simulink model "TempControlExperiment"  (R2016a)
settings: Solver=FixedStepDiscrete  StartTime=0.0  StopTime=inf  FixedStep=1  RelTol=1e-3
libraries: simulink x7, EEE481Arduino x3
settings Model: ExtModeTrigDuration=2  Creator=rsjoshi1  LastModifiedBy=rsjoshi1
settings OptimizationCC: OptimizeModelRefInitCode=on  LifeSpan=Inf  MaxStackSize=64
settings HardwareCC: ProdBitPerPointer=32  ProdLargestAtomicInteger=Long  ProdLargestAtomicFloat=Double  ProdWordSize=32  ProdHWDeviceType=ARM Compatible->ARM Cortex
settings RTWCC: SystemTargetFile=ert.tlc  HardwareBoard=Arduino Due  TemplateMakefile=ert_default_tmf  GenerateReport=on  Toolchain=Arduino ARM v1.6.1  BuildConfiguration=Faster Runs  IncludeHyperlinkInReport=on  LaunchReport=on  GenerateTraceInfo=on  GenerateTraceReport=on  GenerateTraceReportSl=on  GenerateTraceReportSf=on  GenerateTraceReportEml=on
settings CodeAppCC: ForceParamTrailComments=on  IgnoreCustomStorageClasses=off  OperatorAnnotations=on  SimulinkDataObjDesc=on  SFDataObjDesc=on  MATLABFcnDesc=on  InsertBlockDesc=on  MATLABSourceComments=on
settings ERTTargetCC: SupportContinuousTime=on  SupportVariableSizeSignals=on

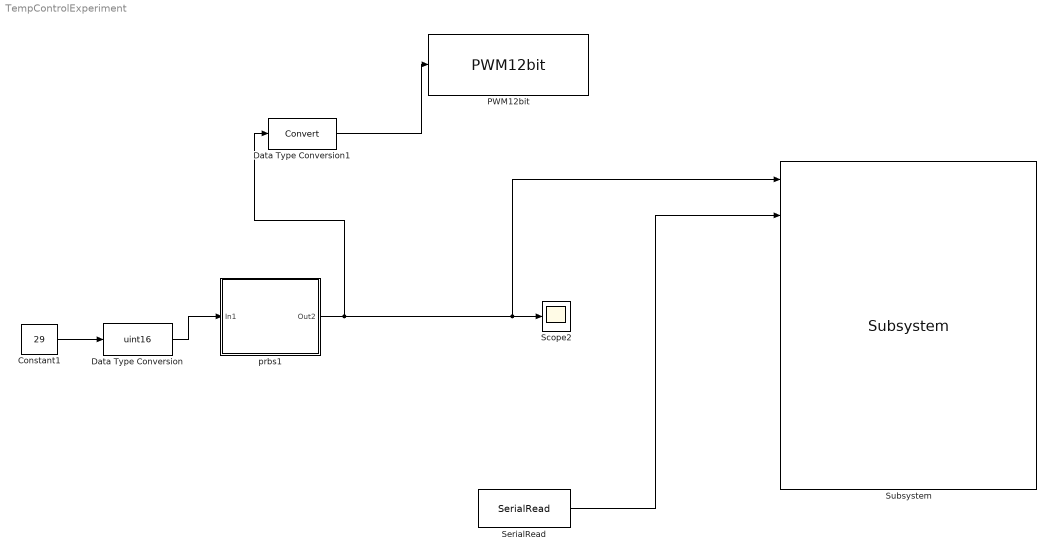
== system TempControlExperiment ==
  Constant1 : Constant  Value=29  OutDataTypeStr=double  SampleTime=1
  Data Type Conversion : DataTypeConversion  OutDataTypeStr=uint16
  Data Type Conversion1 : DataTypeConversion
  PWM12bit : EEE481Arduino/PWM12bit  PwmPort=8
  Scope2 : Scope
  SerialRead : EEE481Arduino/SerialRead  serialNum=2  Ts=1
  Subsystem : EEE481Arduino/Subsystem  Tsa=1  rate=0
  prbs1 : Subsystem
  wires:
  prbs1/1(Out2) -> Data Type Conversion1/1, Subsystem/1, Scope2/1
  Constant1/1 -> Data Type Conversion/1
  Data Type Conversion/1 -> prbs1/1(In1)
  SerialRead/1 -> Subsystem/2
  Data Type Conversion1/1 -> PWM12bit/1

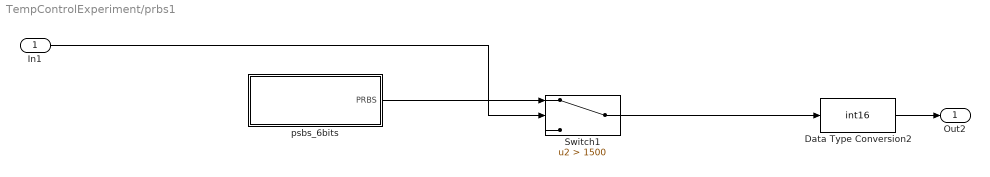
== system TempControlExperiment/prbs1 ==
  In1 : Inport
  Data Type Conversion2 : DataTypeConversion  OutDataTypeStr=int16
  Switch1 : Switch  Criteria=u2 > Threshold  Threshold=1500
  psbs_6bits : Subsystem  mask(PRBS with 8 shift registers){T=-1, Tsw=200, Lz=12000, Lv=60, Nc=100}
      mask prompts: T "Sample Time (s)"; Tsw "Time to switch (s)"; Lz "Leading Zeros (s)"; Lv "Switching Levels"; Nc "Number of Cycles"
      mask help:
      | Creates a PRBS signal using 6 shift registers.
      |     *Time to switch (Tsw) must be an integer multiple of Sample Time (T).
      |     *Leading zeros specify how long the PRBS will be zero, in seconds, before the levels begin shifting.
      |     *Level is the amplitude of the desired PRBS signal. Both + and - levels are equal
      |     *Number of cycles determines the number of full cycles generated. Each cycle is (2^6-1)*Tsw seconds long
  Out2 : Outport
  wires:
  Data Type Conversion2/1 -> Out2/1
  psbs_6bits/1(PRBS) -> Switch1/1
  Switch1/1 -> Data Type Conversion2/1
  In1/1 -> Switch1/2

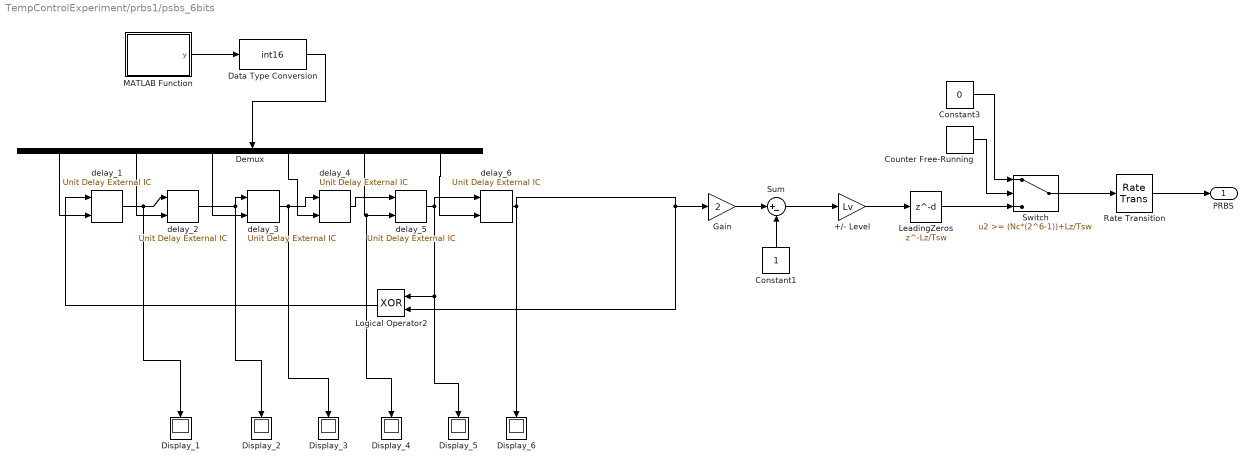
== system TempControlExperiment/prbs1/psbs_6bits ==
  +/- Level : Gain  Gain=Lv  SampleTime=Tsw
  Constant1 : Constant  SampleTime=Tsw
  Constant3 : Constant  Value=0  SampleTime=Tsw
  Counter Free-Running : simulink/Sources/Counter Free-Running  NumBits=32  tsamp=Tsw
  Data Type Conversion : DataTypeConversion  OutDataTypeStr=int16  SampleTime=Tsw
  Demux : Demux  Outputs=6
  Display_{1..6} (6 alike) : Display
  Gain : Gain  Gain=2  SampleTime=Tsw
  LeadingZeros : Delay  DelayLength=Lz/Tsw  InitialCondition=0  SampleTime=Tsw
  Logical Operator2 : Logic  Operator=XOR  AllPortsSameDT=off  OutDataTypeStr=fixdt(1,16)  SampleTime=Tsw
  MATLAB Function : MATLAB Function  TreatAsAtomicUnit=on
  Rate Transition : RateTransition  OutPortSampleTime=T
  Sum : Sum  Inputs=|+-  SampleTime=Tsw
  Switch : Switch  Threshold=(Nc*(2^6-1))+Lz/Tsw  SampleTime=Tsw
  delay_{1..6} (6 alike) : simulink/Additional Math & Discrete/Additional Discrete/Unit Delay External IC  tsamp=Tsw
  PRBS : Outport
  wires:
  delay_5/1 -> Logical Operator2/1, Display_5/1, delay_6/1
  delay_2/1 -> Display_2/1, delay_3/1
  delay_3/1 -> Display_3/1, delay_4/1
  delay_4/1 -> delay_5/1
  delay_1/1 -> delay_2/1, Display_1/1
  delay_6/1 -> Logical Operator2/2, Gain/1, Display_6/1
  MATLAB Function/1(y) -> Data Type Conversion/1
  Demux/6 -> delay_6/2
  Demux/5 -> Display_4/1, delay_5/2
  Demux/4 -> delay_4/2
  Demux/3 -> delay_3/2
  Demux/2 -> delay_2/2
  Demux/1 -> delay_1/2
  Data Type Conversion/1 -> Demux/1
  Sum/1 -> +/- Level/1
  Gain/1 -> Sum/1
  Constant1/1 -> Sum/2
  Logical Operator2/1 -> delay_1/1
  Rate Transition/1 -> PRBS/1
  Counter Free-Running/1 -> Switch/2
  Switch/1 -> Rate Transition/1
  +/- Level/1 -> LeadingZeros/1
  Constant3/1 -> Switch/1
  LeadingZeros/1 -> Switch/3

== matlab function TempControlExperiment/prbs1/psbs_6bits/MATLAB Function ==
  data: y output
function y = fcn()
%#codegen
y = zeros(6,1);
% % s = de2bi(u,16);
% s = dec2bin(u,16);
s = ['1','1','0','1','0','0','1'];
y(1) = s(end-1)-48;
y(2) = s(end-2)-48;
y(3) = s(end-3)-48;
y(4) = s(end-4)-48;
y(5) = s(end-5)-48;
y(6) = s(end-6)-48;
